simulink model "Model"  (R2025b)
settings: Solver=VariableStepAuto  StartTime=0.0  StopTime=10.0  RelTol=1e-3
PreLoadFcn:
  | setup_sim
InitFcn:
  | setup_sim
values from neighbouring files (symbols this model uses):
  hover_throttle = round(exact_throttle)    [setup_sim.m]    (also in setup_sim_PID.m)
undefined symbols (not defined in the file or in its folder): config, DiscIntNeverNeededParam, params
settings Model: Creator=samue  LastModifiedBy=samue

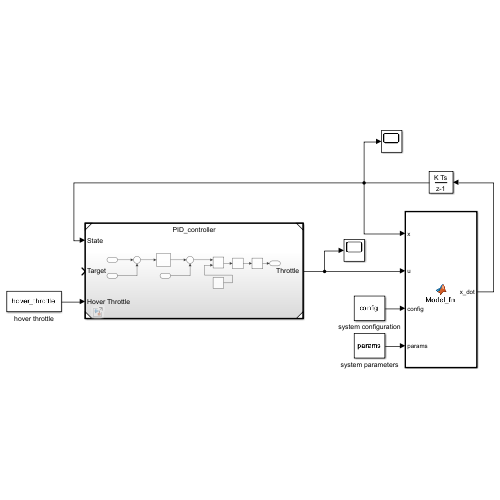
[thumbnail: Simulink's stored preview of the top-level diagram]
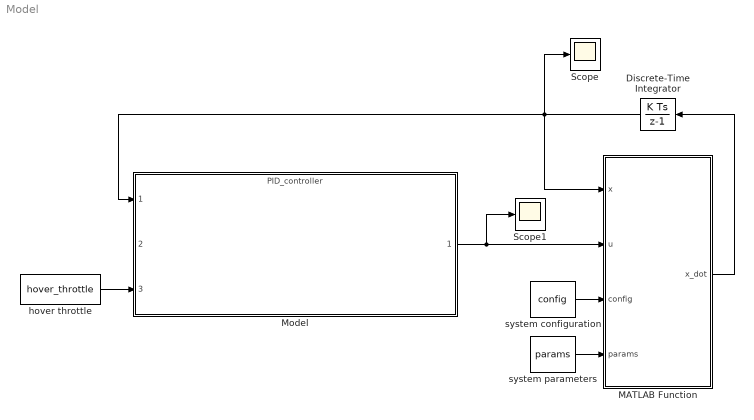
== system Model ==
  Discrete-Time Integrator : DiscreteIntegrator  SampleTime=-1  ICPrevOutput=DiscIntNeverNeededParam  ICPrevScaledInput=DiscIntNeverNeededParam
  MATLAB Function : MATLAB Function  TreatAsAtomicUnit=on
  Model : ModelReference  ModelNameDialog=PID_controller.slx  SimulationMode=Normal  ModelReferenceVersion=1.2
  Scope : Scope
  Scope1 : Scope
  hover throttle : Constant  Value=hover_throttle
  system configuration : Constant  Value=config
  system parameters : Constant  Value=params
  wires:
  system configuration/1 -> MATLAB Function/3(config)
  system parameters/1 -> MATLAB Function/4(params)
  MATLAB Function/1(x_dot) -> Discrete-Time Integrator/1
  Discrete-Time Integrator/1 -> MATLAB Function/1(x), Model/1, Scope/1
  Model/1 -> Scope1/1, MATLAB Function/2(u)
  hover throttle/1 -> Model/3

== matlab function Model/MATLAB Function ==
  data: x input; u input; x_dot output; config input; params input
function x_dot = Model_fn(x, u, config, params)
    x_dot = physics_model(x, u, config, params);
end
